simulink model "Xl_ch16_LPF_int_v6"  (Simulink 7.5)
settings: Solver=VariableStepDiscrete  StartTime=0.0  StopTime=0.001  RelTol=1e-3
values from neighbouring files (symbols this model uses):
  a2a = zeros(nFc, length(Hd.sosMatrix(:,5)))    [iirButter_SOS_init_v2.m]    (also in iirButter_SOS_init_v2_8pole.m)
  a3a = zeros(nFc, length(Hd.sosMatrix(:,6)))    [iirButter_SOS_init_v2.m]    (also in iirButter_SOS_init_v2_8pole.m)
  dt = 1/Fsim    (= 2.56e-06)    [iirButter_SOS_init_v2.m]    (also in iirButter_SOS_init_v2_8pole.m)
  Fc_min = 10    [iirButter_SOS_init_v2.m]    (also in iirButter_SOS_init_v2_8pole.m)
  ga = zeros(nFc, length(Hd.ScaleValues))    [iirButter_SOS_init_v2.m]    (also in iirButter_SOS_init_v2_8pole.m = zeros(nFc, length(Hd.ScaleValues(1:end-1))))
  rFc = (Fc_max/Fc_min)^(1/(nFc - 1))    (= 1.70532863139)    [iirButter_SOS_init_v2.m]    (also in iirButter_SOS_init_v2_8pole.m)
  Sra = 2^34|.02  |.027 |.027 |<.038| 1e-6|<2e-6|<2e-6|<2e-6|<2e-6| 8e-6|    [iirButter_SOS_init_v2.m]    (also in iirButter_SOS_init_v2_8pole.m)
  Srm = 2^34|     |     |     |     |     |     |     |     |     |  to |    [iirButter_SOS_init_v2.m]    (also in iirButter_SOS_init_v2_8pole.m)
libraries: xbsIndex_r4 x561, dspsrcs4 x16, simulink x8
(part 1 of 3)
CloseFcn:
  | rtwprivate ssgencode ModelCloseRequest Xl_ch16_LPF_int_v4
settings Model: Creator=Ivan  LastModifiedBy=val.fleyshman
settings OptimizationCC: InitFltsAndDblsToZero=on
settings DebuggingCC: SaveWithParameterizedLinksMsg=none  SignalResolutionControl=TryResolveAllWithWarning  StrictBusMsg=Warning
settings GRTTargetCC: TargetFcnLib=ansi_tfl_tmw.mat

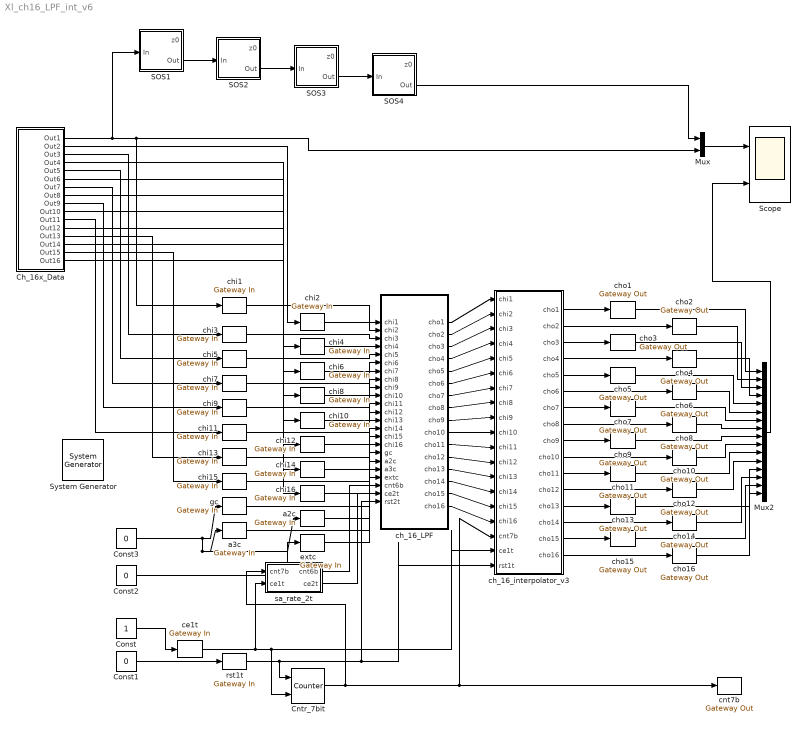
== system Xl_ch16_LPF_int_v6 ==
  " System Generator" : xbsIndex_r4/ System Generator  Tag=genX  SystemSampleTime=-1  xilinxfamily=spartan6  part=xc6slx45t  speed=-3  package=csg324  synthesis_tool=XST  clock_wrapper=Expose Clock Ports  directory=./netlist  testbench=off  simulink_period=1/50e6  sysclk_period=20  dcm_input_clock_period=10  incr_netlist=off  trim_vbits=Everywhere in SubSystem  dbl_ovrd=According to Block Masks  core_generation=According to Block Masks  run_coregen=off  deprecated_control=off  eval_field=0  block_type=sysgen
      settings: block_version=12.2
  Ch_16x_Data : Subsystem
  Cntr_7bit : xbsIndex_r4/Counter  cnt_type=Free Running  cnt_to=Inf  operation=Up  start_count=0  cnt_by_val=1  arith_type=Unsigned  n_bits=7  bin_pt=0  load_pin=off  rst=on  en=on  explicit_period=off  period=1/100e6  dbl_ovrd=off  use_behavioral_HDL=off  implementation=Fabric  block_type=counter
      settings: block_version=12.2
  Const : Constant  OutDataType=sfix(16)  OutScaling=2^0  SampleTime=dt / 128
  Const1 : Constant  Value=0  OutDataType=sfix(16)  OutScaling=2^0  SampleTime=dt / 128
  Const2 : Constant  Value=0  OutDataType=sfix(16)  OutScaling=2^0  SampleTime=dt / 128
  Const3 : Constant  Value=0  OutDataType=sfix(16)  OutScaling=2^0  SampleTime=dt / 128
  Mux : Mux  Inputs=2
  Mux2 : Mux  Inputs=16
  SOS1 : Subsystem
  SOS2 : Subsystem
  SOS3 : Subsystem
  SOS4 : Subsystem
  Scope : Scope  NumInputPorts=2
      settings: YMin=-1~-1  YMax=1~1  DataFormat=Structure  MaxDataPoints=5e6
  a2c : xbsIndex_r4/Gateway In  arith_type="Signed  (2's comp)"  n_bits=36  bin_pt=34  quantization=Truncate  overflow=Wrap  period=1/50e6  dbl_ovrd=off  timing_constraint=None  locs_specified=off  LOCs={}  hdl_port=on  block_type=gatewayin
      settings: infoedit="Gateway in block.  Converts inputs of type Simulink integer, double and fixed point to  Xilinx fixed point type.<br><br>Hardware notes:  In hardware these blocks become top level input ports."  block_version=12.2
  a3c : xbsIndex_r4/Gateway In  arith_type="Signed  (2's comp)"  n_bits=36  bin_pt=34  quantization=Truncate  overflow=Wrap  period=1/50e6  dbl_ovrd=off  timing_constraint=None  locs_specified=off  LOCs={}  hdl_port=on  block_type=gatewayin
      settings: infoedit="Gateway in block.  Converts inputs of type Simulink integer, double and fixed point to  Xilinx fixed point type.<br><br>Hardware notes:  In hardware these blocks become top level input ports."  block_version=12.2
  ce1t : xbsIndex_r4/Gateway In  arith_type=Boolean  n_bits=36  bin_pt=34  quantization=Truncate  overflow=Wrap  period=1/50e6  dbl_ovrd=off  timing_constraint=None  locs_specified=off  LOCs={}  hdl_port=on  block_type=gatewayin
      settings: infoedit="Gateway in block.  Converts inputs of type Simulink integer, double and fixed point to  Xilinx fixed point type.<br><br>Hardware notes:  In hardware these blocks become top level input ports."  block_version=12.2
  ch_16_LPF : Subsystem
  ch_16_interpolator_v3 : Subsystem
  chi{1..16} (16 alike) : xbsIndex_r4/Gateway In  arith_type="Signed  (2's comp)"  n_bits=18  bin_pt=16  quantization=Truncate  overflow=Wrap  period=1/50e6  dbl_ovrd=off  timing_constraint=None  locs_specified=off  LOCs={}  hdl_port=on  block_type=gatewayin
      settings: infoedit="Gateway in block.  Converts inputs of type Simulink integer, double and fixed point to  Xilinx fixed point type.<br><br>Hardware notes:  In hardware these blocks become top level input ports."  block_version=12.2
  cho{1..16} (16 alike) : xbsIndex_r4/Gateway Out  hdl_port=on  timing_constraint=None  locs_specified=off  LOCs={}  block_type=gatewayout
      settings: infoedit="Gateway out block.  Converts Xilinx fixed point inputs into ouputs of type Simulink integer, double, or fixed point.<br><br>Hardware notes:  In hardware these blocks become top level output ports or are discarded, depending on how they are configured."  block_version=12.2
  cnt7b : xbsIndex_r4/Gateway Out  hdl_port=on  timing_constraint=None  locs_specified=off  LOCs={}  block_type=gatewayout
      settings: infoedit="Gateway out block.  Converts Xilinx fixed point inputs into ouputs of type Simulink integer, double, or fixed point.<br><br>Hardware notes:  In hardware these blocks become top level output ports or are discarded, depending on how they are configured."  block_version=12.2
  extc : xbsIndex_r4/Gateway In  arith_type=Boolean  n_bits=36  bin_pt=34  quantization=Truncate  overflow=Wrap  period=1/50e6  dbl_ovrd=off  timing_constraint=None  locs_specified=off  LOCs={}  hdl_port=on  block_type=gatewayin
      settings: infoedit="Gateway in block.  Converts inputs of type Simulink integer, double and fixed point to  Xilinx fixed point type.<br><br>Hardware notes:  In hardware these blocks become top level input ports."  block_version=12.2
  gc : xbsIndex_r4/Gateway In  arith_type="Signed  (2's comp)"  n_bits=36  bin_pt=34  quantization=Truncate  overflow=Wrap  period=1/50e6  dbl_ovrd=off  timing_constraint=None  locs_specified=off  LOCs={}  hdl_port=on  block_type=gatewayin
      settings: infoedit="Gateway in block.  Converts inputs of type Simulink integer, double and fixed point to  Xilinx fixed point type.<br><br>Hardware notes:  In hardware these blocks become top level input ports."  block_version=12.2
  rst1t : xbsIndex_r4/Gateway In  arith_type=Boolean  n_bits=36  bin_pt=34  quantization=Truncate  overflow=Wrap  period=1/50e6  dbl_ovrd=off  timing_constraint=None  locs_specified=off  LOCs={}  hdl_port=on  block_type=gatewayin
      settings: infoedit="Gateway in block.  Converts inputs of type Simulink integer, double and fixed point to  Xilinx fixed point type.<br><br>Hardware notes:  In hardware these blocks become top level input ports."  block_version=12.2
  sa_rate_2t : Subsystem
  wires:
  SOS2/2(Out) -> SOS3/1(In)
  chi1/1 -> ch_16_LPF/1(chi1)
  chi2/1 -> ch_16_LPF/2(chi2)
  chi3/1 -> ch_16_LPF/3(chi3)
  chi4/1 -> ch_16_LPF/4(chi4)
  chi5/1 -> ch_16_LPF/5(chi5)
  chi6/1 -> ch_16_LPF/6(chi6)
  chi7/1 -> ch_16_LPF/7(chi7)
  chi8/1 -> ch_16_LPF/8(chi8)
  chi9/1 -> ch_16_LPF/9(chi9)
  chi10/1 -> ch_16_LPF/10(chi10)
  chi11/1 -> ch_16_LPF/11(chi11)
  chi12/1 -> ch_16_LPF/12(chi12)
  chi13/1 -> ch_16_LPF/13(chi13)
  chi14/1 -> ch_16_LPF/14(chi14)
  chi15/1 -> ch_16_LPF/15(chi15)
  chi16/1 -> ch_16_LPF/16(chi16)
  gc/1 -> ch_16_LPF/17(gc)
  a2c/1 -> ch_16_LPF/18(a2c)
  a3c/1 -> ch_16_LPF/19(a3c)
  ce1t/1 -> sa_rate_2t/2(ce1t), Cntr_7bit/2, ch_16_interpolator_v3/18(ce1t)
  rst1t/1 -> Cntr_7bit/1, ch_16_LPF/23(rst2t), ch_16_interpolator_v3/19(rst1t)
  Const1/1 -> rst1t/1
  sa_rate_2t/2(ce2t) -> ch_16_LPF/22(ce2t)
  extc/1 -> ch_16_LPF/20(extc)
  Const2/1 -> extc/1
  Const3/1 -> gc/1, a3c/1, a2c/1
  Cntr_7bit/1 -> sa_rate_2t/1(cnt7b), cnt7b/1, ch_16_interpolator_v3/17(cnt7b)
  sa_rate_2t/1(cnt6b) -> ch_16_LPF/21(cnt6b)
  Const/1 -> ce1t/1
  Mux/1 -> Scope/1
  SOS3/2(Out) -> SOS4/1(In)
  SOS1/2(Out) -> SOS2/1(In)
  SOS4/2(Out) -> Mux/1
  ch_16_interpolator_v3/1(cho1) -> cho1/1
  ch_16_interpolator_v3/2(cho2) -> cho2/1
  ch_16_interpolator_v3/3(cho3) -> cho3/1
  ch_16_interpolator_v3/4(cho4) -> cho4/1
  ch_16_interpolator_v3/5(cho5) -> cho5/1
  ch_16_interpolator_v3/6(cho6) -> cho6/1
  ch_16_interpolator_v3/7(cho7) -> cho7/1
  ch_16_interpolator_v3/8(cho8) -> cho8/1
  ch_16_interpolator_v3/9(cho9) -> cho9/1
  ch_16_interpolator_v3/10(cho10) -> cho10/1
  ch_16_interpolator_v3/11(cho11) -> cho11/1
  ch_16_interpolator_v3/12(cho12) -> cho12/1
  ch_16_interpolator_v3/13(cho13) -> cho13/1
  ch_16_interpolator_v3/14(cho14) -> cho14/1
  ch_16_interpolator_v3/15(cho15) -> cho15/1
  ch_16_interpolator_v3/16(cho16) -> cho16/1
  cho13/1 -> Mux2/13
  cho1/1 -> Mux2/1
  cho16/1 -> Mux2/16
  cho2/1 -> Mux2/2
  cho3/1 -> Mux2/3
  cho4/1 -> Mux2/4
  cho5/1 -> Mux2/5
  cho6/1 -> Mux2/6
  cho7/1 -> Mux2/7
  cho8/1 -> Mux2/8
  cho9/1 -> Mux2/9
  cho10/1 -> Mux2/10
  cho11/1 -> Mux2/11
  cho12/1 -> Mux2/12
  cho14/1 -> Mux2/14
  cho15/1 -> Mux2/15
  ch_16_LPF/1(cho1) -> ch_16_interpolator_v3/1(chi1)
  ch_16_LPF/2(cho2) -> ch_16_interpolator_v3/2(chi2)
  ch_16_LPF/3(cho3) -> ch_16_interpolator_v3/3(chi3)
  ch_16_LPF/4(cho4) -> ch_16_interpolator_v3/4(chi4)
  ch_16_LPF/5(cho5) -> ch_16_interpolator_v3/5(chi5)
  ch_16_LPF/6(cho6) -> ch_16_interpolator_v3/6(chi6)
  ch_16_LPF/7(cho7) -> ch_16_interpolator_v3/7(chi7)
  ch_16_LPF/8(cho8) -> ch_16_interpolator_v3/8(chi8)
  ch_16_LPF/9(cho9) -> ch_16_interpolator_v3/9(chi9)
  ch_16_LPF/10(cho10) -> ch_16_interpolator_v3/10(chi10)
  ch_16_LPF/11(cho11) -> ch_16_interpolator_v3/11(chi11)
  ch_16_LPF/12(cho12) -> ch_16_interpolator_v3/12(chi12)
  ch_16_LPF/13(cho13) -> ch_16_interpolator_v3/13(chi13)
  ch_16_LPF/14(cho14) -> ch_16_interpolator_v3/14(chi14)
  ch_16_LPF/15(cho15) -> ch_16_interpolator_v3/15(chi15)
  ch_16_LPF/16(cho16) -> ch_16_interpolator_v3/16(chi16)
  Mux2/1 -> Scope/2
  Ch_16x_Data/1(Out1) -> chi1/1, Mux/2, SOS1/1(In)
  Ch_16x_Data/2(Out2) -> chi2/1
  Ch_16x_Data/3(Out3) -> chi3/1
  Ch_16x_Data/4(Out4) -> chi4/1
  Ch_16x_Data/5(Out5) -> chi5/1
  Ch_16x_Data/6(Out6) -> chi6/1
  Ch_16x_Data/7(Out7) -> chi7/1
  Ch_16x_Data/8(Out8) -> chi8/1
  Ch_16x_Data/9(Out9) -> chi9/1
  Ch_16x_Data/10(Out10) -> chi10/1
  Ch_16x_Data/11(Out11) -> chi11/1
  Ch_16x_Data/12(Out12) -> chi12/1
  Ch_16x_Data/13(Out13) -> chi13/1
  Ch_16x_Data/14(Out14) -> chi14/1
  Ch_16x_Data/15(Out15) -> chi15/1
  Ch_16x_Data/16(Out16) -> chi16/1

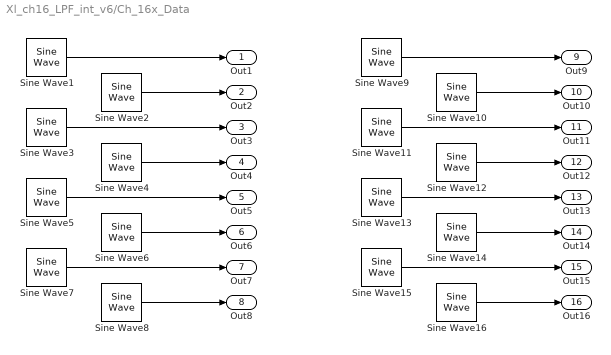
== system Xl_ch16_LPF_int_v6/Ch_16x_Data ==
  Sine Wave1 : dspsrcs4/Sine Wave  Amplitude=1  Frequency=Fc_min * rFc^(1 - 1)  Phase=0  SampleMode=Discrete  OutComplex=Real  CompMethod=Trigonometric fcn  TableSize=Speed  SampleTime=dt  SamplesPerFrame=1  dataType=double  wordLen=16  udDataType=sfix(16)  fracBitsMode=Best precision  numFracBits=15  ResetState=Restart at time zero
  Sine Wave10 : dspsrcs4/Sine Wave  Amplitude=1  Frequency=Fc_min * rFc^(10 - 1)  Phase=0  SampleMode=Discrete  OutComplex=Real  CompMethod=Trigonometric fcn  TableSize=Speed  SampleTime=dt  SamplesPerFrame=1  dataType=double  wordLen=16  udDataType=sfix(16)  fracBitsMode=Best precision  numFracBits=15  ResetState=Restart at time zero
  Sine Wave11 : dspsrcs4/Sine Wave  Amplitude=1  Frequency=Fc_min * rFc^(11 - 1)  Phase=0  SampleMode=Discrete  OutComplex=Real  CompMethod=Trigonometric fcn  TableSize=Speed  SampleTime=dt  SamplesPerFrame=1  dataType=double  wordLen=16  udDataType=sfix(16)  fracBitsMode=Best precision  numFracBits=15  ResetState=Restart at time zero
  Sine Wave12 : dspsrcs4/Sine Wave  Amplitude=1  Frequency=Fc_min * rFc^(12 - 1)  Phase=0  SampleMode=Discrete  OutComplex=Real  CompMethod=Trigonometric fcn  TableSize=Speed  SampleTime=dt  SamplesPerFrame=1  dataType=double  wordLen=16  udDataType=sfix(16)  fracBitsMode=Best precision  numFracBits=15  ResetState=Restart at time zero
  Sine Wave13 : dspsrcs4/Sine Wave  Amplitude=1  Frequency=Fc_min * rFc^(13 - 1)  Phase=0  SampleMode=Discrete  OutComplex=Real  CompMethod=Trigonometric fcn  TableSize=Speed  SampleTime=dt  SamplesPerFrame=1  dataType=double  wordLen=16  udDataType=sfix(16)  fracBitsMode=Best precision  numFracBits=15  ResetState=Restart at time zero
  Sine Wave14 : dspsrcs4/Sine Wave  Amplitude=1  Frequency=Fc_min * rFc^(14 - 1)  Phase=0  SampleMode=Discrete  OutComplex=Real  CompMethod=Trigonometric fcn  TableSize=Speed  SampleTime=dt  SamplesPerFrame=1  dataType=double  wordLen=16  udDataType=sfix(16)  fracBitsMode=Best precision  numFracBits=15  ResetState=Restart at time zero
  Sine Wave15 : dspsrcs4/Sine Wave  Amplitude=1  Frequency=Fc_min * rFc^(15 - 1)  Phase=0  SampleMode=Discrete  OutComplex=Real  CompMethod=Trigonometric fcn  TableSize=Speed  SampleTime=dt  SamplesPerFrame=1  dataType=double  wordLen=16  udDataType=sfix(16)  fracBitsMode=Best precision  numFracBits=15  ResetState=Restart at time zero
  Sine Wave16 : dspsrcs4/Sine Wave  Amplitude=1  Frequency=Fc_min * rFc^(16 - 1)  Phase=0  SampleMode=Discrete  OutComplex=Real  CompMethod=Trigonometric fcn  TableSize=Speed  SampleTime=dt  SamplesPerFrame=1  dataType=double  wordLen=16  udDataType=sfix(16)  fracBitsMode=Best precision  numFracBits=15  ResetState=Restart at time zero
  Sine Wave2 : dspsrcs4/Sine Wave  Amplitude=1  Frequency=Fc_min * rFc^(2 - 1)  Phase=0  SampleMode=Discrete  OutComplex=Real  CompMethod=Trigonometric fcn  TableSize=Speed  SampleTime=dt  SamplesPerFrame=1  dataType=double  wordLen=16  udDataType=sfix(16)  fracBitsMode=Best precision  numFracBits=15  ResetState=Restart at time zero
  Sine Wave3 : dspsrcs4/Sine Wave  Amplitude=1  Frequency=Fc_min * rFc^(3 - 1)  Phase=0  SampleMode=Discrete  OutComplex=Real  CompMethod=Trigonometric fcn  TableSize=Speed  SampleTime=dt  SamplesPerFrame=1  dataType=double  wordLen=16  udDataType=sfix(16)  fracBitsMode=Best precision  numFracBits=15  ResetState=Restart at time zero
  Sine Wave4 : dspsrcs4/Sine Wave  Amplitude=1  Frequency=Fc_min * rFc^(4 - 1)  Phase=0  SampleMode=Discrete  OutComplex=Real  CompMethod=Trigonometric fcn  TableSize=Speed  SampleTime=dt  SamplesPerFrame=1  dataType=double  wordLen=16  udDataType=sfix(16)  fracBitsMode=Best precision  numFracBits=15  ResetState=Restart at time zero
  Sine Wave5 : dspsrcs4/Sine Wave  Amplitude=1  Frequency=Fc_min * rFc^(5 - 1)  Phase=0  SampleMode=Discrete  OutComplex=Real  CompMethod=Trigonometric fcn  TableSize=Speed  SampleTime=dt  SamplesPerFrame=1  dataType=double  wordLen=16  udDataType=sfix(16)  fracBitsMode=Best precision  numFracBits=15  ResetState=Restart at time zero
  Sine Wave6 : dspsrcs4/Sine Wave  Amplitude=1  Frequency=Fc_min * rFc^(6 - 1)  Phase=0  SampleMode=Discrete  OutComplex=Real  CompMethod=Trigonometric fcn  TableSize=Speed  SampleTime=dt  SamplesPerFrame=1  dataType=double  wordLen=16  udDataType=sfix(16)  fracBitsMode=Best precision  numFracBits=15  ResetState=Restart at time zero
  Sine Wave7 : dspsrcs4/Sine Wave  Amplitude=1  Frequency=Fc_min * rFc^(7 - 1)  Phase=0  SampleMode=Discrete  OutComplex=Real  CompMethod=Trigonometric fcn  TableSize=Speed  SampleTime=dt  SamplesPerFrame=1  dataType=double  wordLen=16  udDataType=sfix(16)  fracBitsMode=Best precision  numFracBits=15  ResetState=Restart at time zero
  Sine Wave8 : dspsrcs4/Sine Wave  Amplitude=1  Frequency=Fc_min * rFc^(8 - 1)  Phase=0  SampleMode=Discrete  OutComplex=Real  CompMethod=Trigonometric fcn  TableSize=Speed  SampleTime=dt  SamplesPerFrame=1  dataType=double  wordLen=16  udDataType=sfix(16)  fracBitsMode=Best precision  numFracBits=15  ResetState=Restart at time zero
  Sine Wave9 : dspsrcs4/Sine Wave  Amplitude=1  Frequency=Fc_min * rFc^(9 - 1)  Phase=0  SampleMode=Discrete  OutComplex=Real  CompMethod=Trigonometric fcn  TableSize=Speed  SampleTime=dt  SamplesPerFrame=1  dataType=double  wordLen=16  udDataType=sfix(16)  fracBitsMode=Best precision  numFracBits=15  ResetState=Restart at time zero
  Out1 : Outport
  Out2 : Outport  Port=2
  Out3 : Outport  Port=3
  Out4 : Outport  Port=4
  Out5 : Outport  Port=5
  Out6 : Outport  Port=6
  Out7 : Outport  Port=7
  Out8 : Outport  Port=8
  Out9 : Outport  Port=9
  Out10 : Outport  Port=10
  Out11 : Outport  Port=11
  Out12 : Outport  Port=12
  Out13 : Outport  Port=13
  Out14 : Outport  Port=14
  Out15 : Outport  Port=15
  Out16 : Outport  Port=16
  wires:
  Sine Wave16/1 -> Out16/1
  Sine Wave15/1 -> Out15/1
  Sine Wave14/1 -> Out14/1
  Sine Wave13/1 -> Out13/1
  Sine Wave12/1 -> Out12/1
  Sine Wave11/1 -> Out11/1
  Sine Wave10/1 -> Out10/1
  Sine Wave9/1 -> Out9/1
  Sine Wave8/1 -> Out8/1
  Sine Wave7/1 -> Out7/1
  Sine Wave6/1 -> Out6/1
  Sine Wave5/1 -> Out5/1
  Sine Wave4/1 -> Out4/1
  Sine Wave3/1 -> Out3/1
  Sine Wave2/1 -> Out2/1
  Sine Wave1/1 -> Out1/1

== system Xl_ch16_LPF_int_v6/SOS1 ==
  note: b1 = 1
  note: b3 = 1
  note: 1/a1 = 1
  In : Inport
  Delay : simulink/Discrete/Integer Delay  vinit=0.0  samptime=-1  NumDelays=1
  Delay1 : simulink/Discrete/Integer Delay  vinit=0.0  samptime=-1  NumDelays=1
  Round RA : Subsystem
  Round RA1 : Subsystem
  Round RM : Subsystem
  Round RM1 : Subsystem
  Round RM2 : Subsystem
  Sum Denom1 : Sum  Inputs=+-  OutDataType=sfix(16)  OutScaling=2^0
  Sum Denom2 : Sum  Inputs=+-  OutDataType=sfix(16)  OutScaling=2^0
  Sum Num1 : Sum  OutDataType=sfix(16)  OutScaling=2^0
  Sum Num2 : Sum  OutDataType=sfix(16)  OutScaling=2^0
  a2 : Gain  Gain=a2a(13,1)  ParameterDataType=sfix(16)  ParameterScaling=2^0  OutDataType=sfix(16)  OutScaling=2^0
  a3 : Gain  Gain=a3a(13,1)  ParameterDataType=sfix(16)  ParameterScaling=2^0  OutDataType=sfix(16)  OutScaling=2^0
  b2 : Gain  Gain=2  ParameterDataType=sfix(16)  ParameterScaling=2^0  OutDataType=sfix(16)  OutScaling=2^0
  g : Gain  Gain=ga(13,1)  ParameterDataType=sfix(16)  ParameterScaling=2^0  OutDataType=sfix(16)  OutScaling=2^0
  z0 : Outport
  Out : Outport  Port=2
  wires:
  Delay/1 -> Delay1/1, b2/1, a2/1
  b2/1 -> Sum Num1/2
  Delay1/1 -> a3/1, Sum Num2/2
  Sum Denom2/1 -> Round RA/1(In)
  a2/1 -> Round RM1/1(In)
  a3/1 -> Round RM2/1(In)
  g/1 -> Round RM/1(In)
  In/1 -> g/1
  Sum Num2/1 -> Round RA1/1(In)
  Round RM/1(Out) -> Sum Denom1/1
  Round RA/1(Out) -> Delay/1, z0/1, Sum Num1/1
  Round RA1/1(Out) -> Out/1
  Sum Num1/1 -> Sum Num2/1
  Sum Denom1/1 -> Sum Denom2/1
  Round RM1/1(Out) -> Sum Denom1/2
  Round RM2/1(Out) -> Sum Denom2/2

== system Xl_ch16_LPF_int_v6/SOS2 ==
  note: 1/a1 = 1
  note: b3 = 1
  note: b1 = 1
  In : Inport
  Delay : simulink/Discrete/Integer Delay  vinit=0.0  samptime=-1  NumDelays=1
  Delay1 : simulink/Discrete/Integer Delay  vinit=0.0  samptime=-1  NumDelays=1
  Round RA : Subsystem
  Round RA1 : Subsystem
  Round RM : Subsystem
  Round RM1 : Subsystem
  Round RM2 : Subsystem
  Sum Denom1 : Sum  Inputs=+-  OutDataType=sfix(16)  OutScaling=2^0
  Sum Denom2 : Sum  Inputs=+-  OutDataType=sfix(16)  OutScaling=2^0
  Sum Num1 : Sum  OutDataType=sfix(16)  OutScaling=2^0
  Sum Num2 : Sum  OutDataType=sfix(16)  OutScaling=2^0
  a2 : Gain  Gain=a2a(13,2)  ParameterDataType=sfix(16)  ParameterScaling=2^0  OutDataType=sfix(16)  OutScaling=2^0
  a3 : Gain  Gain=a3a(13,2)  ParameterDataType=sfix(16)  ParameterScaling=2^0  OutDataType=sfix(16)  OutScaling=2^0
  b2 : Gain  Gain=2  ParameterDataType=sfix(16)  ParameterScaling=2^0  OutDataType=sfix(16)  OutScaling=2^0
  g : Gain  Gain=ga(13,2)  ParameterDataType=sfix(16)  ParameterScaling=2^0  OutDataType=sfix(16)  OutScaling=2^0
  z0 : Outport
  Out : Outport  Port=2
  wires:
  Round RM2/1(Out) -> Sum Denom2/2
  Round RM1/1(Out) -> Sum Denom1/2
  Sum Denom1/1 -> Sum Denom2/1
  Sum Num1/1 -> Sum Num2/1
  Round RA1/1(Out) -> Out/1
  Round RA/1(Out) -> Sum Num1/1, z0/1, Delay/1
  Round RM/1(Out) -> Sum Denom1/1
  Sum Num2/1 -> Round RA1/1(In)
  In/1 -> g/1
  g/1 -> Round RM/1(In)
  a3/1 -> Round RM2/1(In)
  a2/1 -> Round RM1/1(In)
  Sum Denom2/1 -> Round RA/1(In)
  Delay1/1 -> Sum Num2/2, a3/1
  b2/1 -> Sum Num1/2
  Delay/1 -> a2/1, b2/1, Delay1/1

== system Xl_ch16_LPF_int_v6/SOS3 ==
  note: b1 = 1
  note: b3 = 1
  note: 1/a1 = 1
  In : Inport
  Delay : simulink/Discrete/Integer Delay  vinit=0.0  samptime=-1  NumDelays=1
  Delay1 : simulink/Discrete/Integer Delay  vinit=0.0  samptime=-1  NumDelays=1
  Round RA : Subsystem
  Round RA1 : Subsystem
  Round RM : Subsystem
  Round RM1 : Subsystem
  Round RM2 : Subsystem
  Sum Denom1 : Sum  Inputs=+-  OutDataType=sfix(16)  OutScaling=2^0
  Sum Denom2 : Sum  Inputs=+-  OutDataType=sfix(16)  OutScaling=2^0
  Sum Num1 : Sum  OutDataType=sfix(16)  OutScaling=2^0
  Sum Num2 : Sum  OutDataType=sfix(16)  OutScaling=2^0
  a2 : Gain  Gain=a2a(13,3)  ParameterDataType=sfix(16)  ParameterScaling=2^0  OutDataType=sfix(16)  OutScaling=2^0
  a3 : Gain  Gain=a3a(13,3)  ParameterDataType=sfix(16)  ParameterScaling=2^0  OutDataType=sfix(16)  OutScaling=2^0
  b2 : Gain  Gain=2  ParameterDataType=sfix(16)  ParameterScaling=2^0  OutDataType=sfix(16)  OutScaling=2^0
  g : Gain  Gain=ga(13,3)  ParameterDataType=sfix(16)  ParameterScaling=2^0  OutDataType=sfix(16)  OutScaling=2^0
  z0 : Outport
  Out : Outport  Port=2
  wires:
  Delay/1 -> Delay1/1, b2/1, a2/1
  b2/1 -> Sum Num1/2
  Delay1/1 -> a3/1, Sum Num2/2
  Sum Denom2/1 -> Round RA/1(In)
  a2/1 -> Round RM1/1(In)
  a3/1 -> Round RM2/1(In)
  g/1 -> Round RM/1(In)
  In/1 -> g/1
  Sum Num2/1 -> Round RA1/1(In)
  Round RM/1(Out) -> Sum Denom1/1
  Round RA/1(Out) -> Delay/1, z0/1, Sum Num1/1
  Round RA1/1(Out) -> Out/1
  Sum Num1/1 -> Sum Num2/1
  Sum Denom1/1 -> Sum Denom2/1
  Round RM1/1(Out) -> Sum Denom1/2
  Round RM2/1(Out) -> Sum Denom2/2

== system Xl_ch16_LPF_int_v6/SOS4 ==
  note: b1 = 1
  note: b3 = 1
  note: 1/a1 = 1
  In : Inport
  Delay : simulink/Discrete/Integer Delay  vinit=0.0  samptime=-1  NumDelays=1
  Delay1 : simulink/Discrete/Integer Delay  vinit=0.0  samptime=-1  NumDelays=1
  Round RA : Subsystem
  Round RA1 : Subsystem
  Round RM : Subsystem
  Round RM1 : Subsystem
  Round RM2 : Subsystem
  Sum Denom1 : Sum  Inputs=+-  OutDataType=sfix(16)  OutScaling=2^0
  Sum Denom2 : Sum  Inputs=+-  OutDataType=sfix(16)  OutScaling=2^0
  Sum Num1 : Sum  OutDataType=sfix(16)  OutScaling=2^0
  Sum Num2 : Sum  OutDataType=sfix(16)  OutScaling=2^0
  a2 : Gain  Gain=a2a(13,4)  ParameterDataType=sfix(16)  ParameterScaling=2^0  OutDataType=sfix(16)  OutScaling=2^0
  a3 : Gain  Gain=a3a(13,4)  ParameterDataType=sfix(16)  ParameterScaling=2^0  OutDataType=sfix(16)  OutScaling=2^0
  b2 : Gain  Gain=2  ParameterDataType=sfix(16)  ParameterScaling=2^0  OutDataType=sfix(16)  OutScaling=2^0
  g : Gain  Gain=ga(13,4)  ParameterDataType=sfix(16)  ParameterScaling=2^0  OutDataType=sfix(16)  OutScaling=2^0
  z0 : Outport
  Out : Outport  Port=2
  wires:
  Delay/1 -> Delay1/1, b2/1, a2/1
  b2/1 -> Sum Num1/2
  Delay1/1 -> a3/1, Sum Num2/2
  Sum Denom2/1 -> Round RA/1(In)
  a2/1 -> Round RM1/1(In)
  a3/1 -> Round RM2/1(In)
  g/1 -> Round RM/1(In)
  In/1 -> g/1
  Sum Num2/1 -> Round RA1/1(In)
  Round RM/1(Out) -> Sum Denom1/1
  Round RA/1(Out) -> Delay/1, z0/1, Sum Num1/1
  Round RA1/1(Out) -> Out/1
  Sum Num1/1 -> Sum Num2/1
  Sum Denom1/1 -> Sum Denom2/1
  Round RM1/1(Out) -> Sum Denom1/2
  Round RM2/1(Out) -> Sum Denom2/2

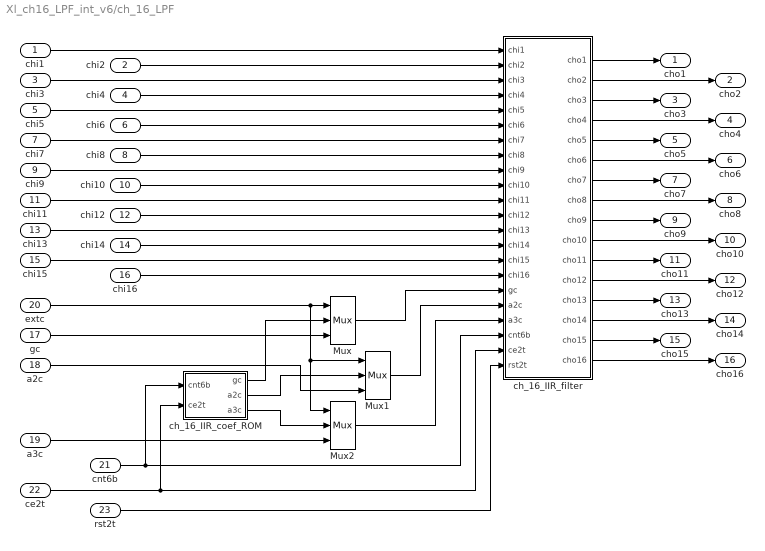
== system Xl_ch16_LPF_int_v6/ch_16_LPF ==
  chi1 : Inport
  chi2 : Inport  Port=2
  chi3 : Inport  Port=3
  chi4 : Inport  Port=4
  chi5 : Inport  Port=5
  chi6 : Inport  Port=6
  chi7 : Inport  Port=7
  chi8 : Inport  Port=8
  chi9 : Inport  Port=9
  chi10 : Inport  Port=10
  chi11 : Inport  Port=11
  chi12 : Inport  Port=12
  chi13 : Inport  Port=13
  chi14 : Inport  Port=14
  chi15 : Inport  Port=15
  chi16 : Inport  Port=16
  gc : Inport  Port=17
  a2c : Inport  Port=18
  a3c : Inport  Port=19
  extc : Inport  Port=20
  cnt6b : Inport  Port=21
  ce2t : Inport  Port=22
  rst2t : Inport  Port=23
  Mux : xbsIndex_r4/Mux  inputs=2  en=off  latency=0  precision=Full  arith_type=Unsigned  n_bits=16  bin_pt=14  quantization=Truncate  overflow=Wrap  dbl_ovrd=off  block_type=mux
      settings: block_version=12.2
  Mux1 : xbsIndex_r4/Mux  inputs=2  en=off  latency=0  precision=Full  arith_type=Unsigned  n_bits=16  bin_pt=14  quantization=Truncate  overflow=Wrap  dbl_ovrd=off  block_type=mux
      settings: block_version=12.2
  Mux2 : xbsIndex_r4/Mux  inputs=2  en=off  latency=0  precision=Full  arith_type=Unsigned  n_bits=16  bin_pt=14  quantization=Truncate  overflow=Wrap  dbl_ovrd=off  block_type=mux
      settings: block_version=12.2
  ch_16_IIR_coef_ROM : Subsystem
  ch_16_IIR_filter : Subsystem
  cho1 : Outport
  cho2 : Outport  Port=2
  cho3 : Outport  Port=3
  cho4 : Outport  Port=4
  cho5 : Outport  Port=5
  cho6 : Outport  Port=6
  cho7 : Outport  Port=7
  cho8 : Outport  Port=8
  cho9 : Outport  Port=9
  cho10 : Outport  Port=10
  cho11 : Outport  Port=11
  cho12 : Outport  Port=12
  cho13 : Outport  Port=13
  cho14 : Outport  Port=14
  cho15 : Outport  Port=15
  cho16 : Outport  Port=16
  wires:
  chi1/1 -> ch_16_IIR_filter/1(chi1)
  ch_16_IIR_filter/1(cho1) -> cho1/1
  chi2/1 -> ch_16_IIR_filter/2(chi2)
  ch_16_IIR_filter/2(cho2) -> cho2/1
  chi3/1 -> ch_16_IIR_filter/3(chi3)
  ch_16_IIR_filter/3(cho3) -> cho3/1
  chi4/1 -> ch_16_IIR_filter/4(chi4)
  chi5/1 -> ch_16_IIR_filter/5(chi5)
  ch_16_IIR_filter/4(cho4) -> cho4/1
  chi6/1 -> ch_16_IIR_filter/6(chi6)
  ch_16_IIR_filter/5(cho5) -> cho5/1
  chi7/1 -> ch_16_IIR_filter/7(chi7)
  ch_16_IIR_filter/6(cho6) -> cho6/1
  chi8/1 -> ch_16_IIR_filter/8(chi8)
  chi9/1 -> ch_16_IIR_filter/9(chi9)
  ch_16_IIR_filter/7(cho7) -> cho7/1
  chi10/1 -> ch_16_IIR_filter/10(chi10)
  ch_16_IIR_filter/8(cho8) -> cho8/1
  chi11/1 -> ch_16_IIR_filter/11(chi11)
  ch_16_IIR_filter/9(cho9) -> cho9/1
  chi12/1 -> ch_16_IIR_filter/12(chi12)
  chi13/1 -> ch_16_IIR_filter/13(chi13)
  ch_16_IIR_filter/10(cho10) -> cho10/1
  chi14/1 -> ch_16_IIR_filter/14(chi14)
  ch_16_IIR_filter/11(cho11) -> cho11/1
  chi15/1 -> ch_16_IIR_filter/15(chi15)
  ch_16_IIR_filter/12(cho12) -> cho12/1
  chi16/1 -> ch_16_IIR_filter/16(chi16)
  ch_16_IIR_filter/13(cho13) -> cho13/1
  ch_16_IIR_filter/14(cho14) -> cho14/1
  ch_16_IIR_filter/15(cho15) -> cho15/1
  ce2t/1 -> ch_16_IIR_coef_ROM/2(ce2t), ch_16_IIR_filter/21(ce2t)
  ch_16_IIR_filter/16(cho16) -> cho16/1
  gc/1 -> Mux/3
  Mux/1 -> ch_16_IIR_filter/17(gc)
  a2c/1 -> Mux1/3
  Mux1/1 -> ch_16_IIR_filter/18(a2c)
  Mux2/1 -> ch_16_IIR_filter/19(a3c)
  a3c/1 -> Mux2/3
  extc/1 -> Mux/1, Mux2/1, Mux1/1
  ch_16_IIR_coef_ROM/1(gc) -> Mux/2
  ch_16_IIR_coef_ROM/3(a3c) -> Mux2/2
  rst2t/1 -> ch_16_IIR_filter/22(rst2t)
  cnt6b/1 -> ch_16_IIR_coef_ROM/1(cnt6b), ch_16_IIR_filter/20(cnt6b)
  ch_16_IIR_coef_ROM/2(a2c) -> Mux1/2

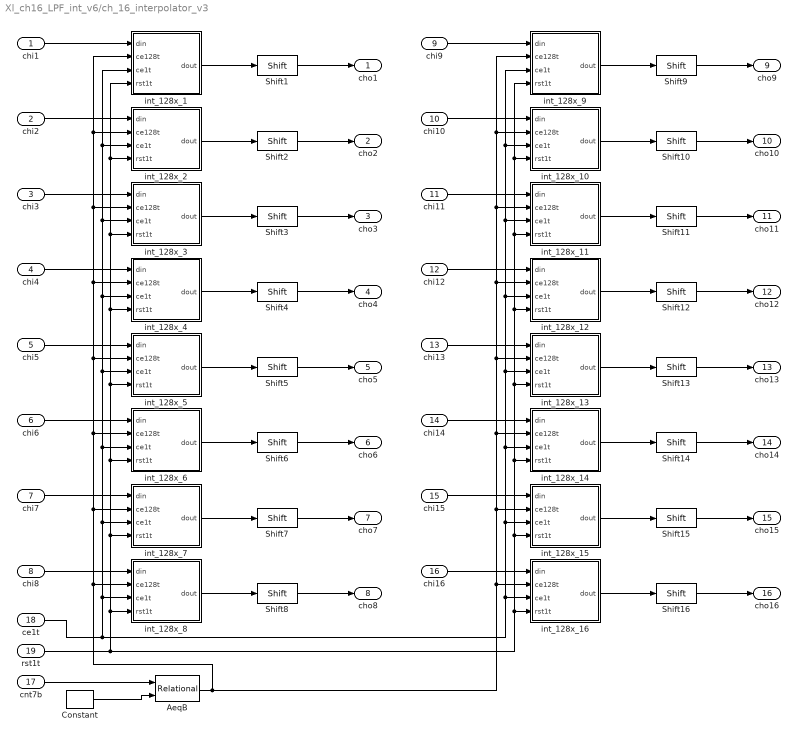
== system Xl_ch16_LPF_int_v6/ch_16_interpolator_v3 ==
  chi1 : Inport
  chi2 : Inport  Port=2
  chi3 : Inport  Port=3
  chi4 : Inport  Port=4
  chi5 : Inport  Port=5
  chi6 : Inport  Port=6
  chi7 : Inport  Port=7
  chi8 : Inport  Port=8
  chi9 : Inport  Port=9
  chi10 : Inport  Port=10
  chi11 : Inport  Port=11
  chi12 : Inport  Port=12
  chi13 : Inport  Port=13
  chi14 : Inport  Port=14
  chi15 : Inport  Port=15
  chi16 : Inport  Port=16
  cnt7b : Inport  Port=17
  ce1t : Inport  Port=18
  rst1t : Inport  Port=19
  AeqB : xbsIndex_r4/Relational  mode=a=b  en=off  latency=0  dbl_ovrd=off  block_type=relational
      settings: block_version=12.2
  Constant : xbsIndex_r4/Constant  arith_type=Unsigned  const=0  n_bits=7  bin_pt=0  explicit_period=off  period=1  equ=P=C  opselect=C  inp2=PCIN>>17  opr=+  inp1=P  carry=CIN  dbl_ovrd=off  block_type=constant
      settings: block_version=12.2
  Shift{1..16} (16 alike) : xbsIndex_r4/Shift  shift_dir=Right  shift_bits=14  en=off  latency=0  precision=User Defined  arith_type="Signed  (2's comp)"  n_bits=18  bin_pt=16  quantization=Truncate  overflow=Wrap  dbl_ovrd=off  block_type=shift
      settings: xl_area=[0 0 0 0 0 0 0]  block_version=12.2
  int_128x_1 : Subsystem
  int_128x_10 : Subsystem
  int_128x_11 : Subsystem
  int_128x_12 : Subsystem
  int_128x_13 : Subsystem
  int_128x_14 : Subsystem
  int_128x_15 : Subsystem
  int_128x_16 : Subsystem
  int_128x_2 : Subsystem
  int_128x_3 : Subsystem
  int_128x_4 : Subsystem
  int_128x_5 : Subsystem
  int_128x_6 : Subsystem
  int_128x_7 : Subsystem
  int_128x_8 : Subsystem
  int_128x_9 : Subsystem
  cho1 : Outport
  cho2 : Outport  Port=2
  cho3 : Outport  Port=3
  cho4 : Outport  Port=4
  cho5 : Outport  Port=5
  cho6 : Outport  Port=6
  cho7 : Outport  Port=7
  cho8 : Outport  Port=8
  cho9 : Outport  Port=9
  cho10 : Outport  Port=10
  cho11 : Outport  Port=11
  cho12 : Outport  Port=12
  cho13 : Outport  Port=13
  cho14 : Outport  Port=14
  cho15 : Outport  Port=15
  cho16 : Outport  Port=16
  wires:
  int_128x_1/1(dout) -> Shift1/1
  chi1/1 -> int_128x_1/1(din)
  Shift1/1 -> cho1/1
  int_128x_2/1(dout) -> Shift2/1
  chi2/1 -> int_128x_2/1(din)
  Shift2/1 -> cho2/1
  int_128x_3/1(dout) -> Shift3/1
  chi3/1 -> int_128x_3/1(din)
  Shift3/1 -> cho3/1
  int_128x_4/1(dout) -> Shift4/1
  chi4/1 -> int_128x_4/1(din)
  Shift4/1 -> cho4/1
  int_128x_5/1(dout) -> Shift5/1
  chi5/1 -> int_128x_5/1(din)
  Shift5/1 -> cho5/1
  int_128x_6/1(dout) -> Shift6/1
  chi6/1 -> int_128x_6/1(din)
  Shift6/1 -> cho6/1
  int_128x_7/1(dout) -> Shift7/1
  chi7/1 -> int_128x_7/1(din)
  Shift7/1 -> cho7/1
  int_128x_8/1(dout) -> Shift8/1
  chi8/1 -> int_128x_8/1(din)
  Shift8/1 -> cho8/1
  int_128x_9/1(dout) -> Shift9/1
  chi9/1 -> int_128x_9/1(din)
  Shift9/1 -> cho9/1
  int_128x_10/1(dout) -> Shift10/1
  chi10/1 -> int_128x_10/1(din)
  Shift10/1 -> cho10/1
  int_128x_11/1(dout) -> Shift11/1
  chi11/1 -> int_128x_11/1(din)
  Shift11/1 -> cho11/1
  int_128x_12/1(dout) -> Shift12/1
  chi12/1 -> int_128x_12/1(din)
  Shift12/1 -> cho12/1
  int_128x_13/1(dout) -> Shift13/1
  chi13/1 -> int_128x_13/1(din)
  Shift13/1 -> cho13/1
  int_128x_14/1(dout) -> Shift14/1
  chi14/1 -> int_128x_14/1(din)
  Shift14/1 -> cho14/1
  int_128x_15/1(dout) -> Shift15/1
  chi15/1 -> int_128x_15/1(din)
  Shift15/1 -> cho15/1
  int_128x_16/1(dout) -> Shift16/1
  chi16/1 -> int_128x_16/1(din)
  Shift16/1 -> cho16/1
  rst1t/1 -> int_128x_1/4(rst1t), int_128x_2/4(rst1t), int_128x_3/4(rst1t), int_128x_4/4(rst1t), int_128x_5/4(rst1t), int_128x_6/4(rst1t), int_128x_7/4(rst1t), int_128x_8/4(rst1t), int_128x_9/4(rst1t), int_128x_10/4(rst1t), int_128x_11/4(rst1t), int_128x_12/4(rst1t), int_128x_13/4(rst1t), int_128x_14/4(rst1t), int_128x_15/4(rst1t), int_128x_16/4(rst1t)
  ce1t/1 -> int_128x_1/3(ce1t), int_128x_2/3(ce1t), int_128x_3/3(ce1t), int_128x_4/3(ce1t), int_128x_5/3(ce1t), int_128x_6/3(ce1t), int_128x_7/3(ce1t), int_128x_8/3(ce1t), int_128x_9/3(ce1t), int_128x_10/3(ce1t), int_128x_11/3(ce1t), int_128x_12/3(ce1t), int_128x_13/3(ce1t), int_128x_14/3(ce1t), int_128x_15/3(ce1t), int_128x_16/3(ce1t)
  AeqB/1 -> int_128x_1/2(ce128t), int_128x_2/2(ce128t), int_128x_3/2(ce128t), int_128x_4/2(ce128t), int_128x_5/2(ce128t), int_128x_6/2(ce128t), int_128x_7/2(ce128t), int_128x_8/2(ce128t), int_128x_9/2(ce128t), int_128x_10/2(ce128t), int_128x_11/2(ce128t), int_128x_12/2(ce128t), int_128x_13/2(ce128t), int_128x_14/2(ce128t), int_128x_15/2(ce128t), int_128x_16/2(ce128t)
  cnt7b/1 -> AeqB/1
  Constant/1 -> AeqB/2

== system Xl_ch16_LPF_int_v6/sa_rate_2t ==
  cnt7b : Inport
  ce1t : Inport  Port=2
  Extract_LSB : xbsIndex_r4/Slice  nbits=1  boolean_output=on  mode=Lower Bit Location + Width  bit1=0  base1=MSB of Input  bit0=0  base0=LSB of Input  dbl_ovrd=off  block_type=slice
      settings: block_version=12.2
  Logical : xbsIndex_r4/Logical  logical_function=AND  inputs=2  en=off  latency=0  precision=Full  arith_type=Unsigned  n_bits=16  bin_pt=0  align_bp=on  dbl_ovrd=off  block_type=logical
      settings: block_version=12.2
  Slice_6MSB : xbsIndex_r4/Slice  nbits=6  boolean_output=off  mode=Upper Bit Location + Width  bit1=0  base1=MSB of Input  bit0=0  base0=LSB of Input  dbl_ovrd=off  block_type=slice
      settings: block_version=12.2
  cnt6b : Outport
  ce2t : Outport  Port=2
  wires:
  cnt7b/1 -> Slice_6MSB/1, Extract_LSB/1
  Slice_6MSB/1 -> cnt6b/1
  Extract_LSB/1 -> Logical/1
  Logical/1 -> ce2t/1
  ce1t/1 -> Logical/2

== system Xl_ch16_LPF_int_v6/SOS1/Round RA ==
  In : Inport
  Rounding Function : Rounding  Operator=round
  Scale Back : Gain  Gain=1/Sra  ParameterDataType=sfix(16)  ParameterScaling=2^0  OutDataType=sfix(16)  OutScaling=2^0
  Scale Up : Gain  Gain=Sra  ParameterDataType=sfix(16)  ParameterScaling=2^0  OutDataType=sfix(16)  OutScaling=2^0
  Out : Outport
  wires:
  Scale Back/1 -> Out/1
  In/1 -> Scale Up/1
  Rounding Function/1 -> Scale Back/1
  Scale Up/1 -> Rounding Function/1

== system Xl_ch16_LPF_int_v6/SOS1/Round RA1 ==
  In : Inport
  Rounding Function : Rounding  Operator=round
  Scale Back : Gain  Gain=1/Sra  ParameterDataType=sfix(16)  ParameterScaling=2^0  OutDataType=sfix(16)  OutScaling=2^0
  Scale Up : Gain  Gain=Sra  ParameterDataType=sfix(16)  ParameterScaling=2^0  OutDataType=sfix(16)  OutScaling=2^0
  Out : Outport
  wires:
  Scale Up/1 -> Rounding Function/1
  Rounding Function/1 -> Scale Back/1
  In/1 -> Scale Up/1
  Scale Back/1 -> Out/1

== system Xl_ch16_LPF_int_v6/SOS1/Round RM ==
  In : Inport
  Rounding Function : Rounding  Operator=round
  Scale Back : Gain  Gain=1/Srm  ParameterDataType=sfix(16)  ParameterScaling=2^0  OutDataType=sfix(16)  OutScaling=2^0
  Scale Up : Gain  Gain=Srm  ParameterDataType=sfix(16)  ParameterScaling=2^0  OutDataType=sfix(16)  OutScaling=2^0
  Out : Outport
  wires:
  Scale Up/1 -> Rounding Function/1
  Rounding Function/1 -> Scale Back/1
  In/1 -> Scale Up/1
  Scale Back/1 -> Out/1

== system Xl_ch16_LPF_int_v6/SOS1/Round RM1 ==
  In : Inport
  Rounding Function : Rounding  Operator=round
  Scale Back : Gain  Gain=1/Srm  ParameterDataType=sfix(16)  ParameterScaling=2^0  OutDataType=sfix(16)  OutScaling=2^0
  Scale Up : Gain  Gain=Srm  ParameterDataType=sfix(16)  ParameterScaling=2^0  OutDataType=sfix(16)  OutScaling=2^0
  Out : Outport
  wires:
  Scale Back/1 -> Out/1
  In/1 -> Scale Up/1
  Rounding Function/1 -> Scale Back/1
  Scale Up/1 -> Rounding Function/1

== system Xl_ch16_LPF_int_v6/SOS1/Round RM2 ==
  In : Inport
  Rounding Function : Rounding  Operator=round
  Scale Back : Gain  Gain=1/Srm  ParameterDataType=sfix(16)  ParameterScaling=2^0  OutDataType=sfix(16)  OutScaling=2^0
  Scale Up : Gain  Gain=Srm  ParameterDataType=sfix(16)  ParameterScaling=2^0  OutDataType=sfix(16)  OutScaling=2^0
  Out : Outport
  wires:
  Scale Up/1 -> Rounding Function/1
  Rounding Function/1 -> Scale Back/1
  In/1 -> Scale Up/1
  Scale Back/1 -> Out/1

== system Xl_ch16_LPF_int_v6/SOS2/Round RA ==
  In : Inport
  Rounding Function : Rounding  Operator=round
  Scale Back : Gain  Gain=1/Sra  ParameterDataType=sfix(16)  ParameterScaling=2^0  OutDataType=sfix(16)  OutScaling=2^0
  Scale Up : Gain  Gain=Sra  ParameterDataType=sfix(16)  ParameterScaling=2^0  OutDataType=sfix(16)  OutScaling=2^0
  Out : Outport
  wires:
  Scale Up/1 -> Rounding Function/1
  Rounding Function/1 -> Scale Back/1
  In/1 -> Scale Up/1
  Scale Back/1 -> Out/1

== system Xl_ch16_LPF_int_v6/SOS2/Round RA1 ==
  In : Inport
  Rounding Function : Rounding  Operator=round
  Scale Back : Gain  Gain=1/Sra  ParameterDataType=sfix(16)  ParameterScaling=2^0  OutDataType=sfix(16)  OutScaling=2^0
  Scale Up : Gain  Gain=Sra  ParameterDataType=sfix(16)  ParameterScaling=2^0  OutDataType=sfix(16)  OutScaling=2^0
  Out : Outport
  wires:
  Scale Back/1 -> Out/1
  In/1 -> Scale Up/1
  Rounding Function/1 -> Scale Back/1
  Scale Up/1 -> Rounding Function/1

== system Xl_ch16_LPF_int_v6/SOS2/Round RM ==
  In : Inport
  Rounding Function : Rounding  Operator=round
  Scale Back : Gain  Gain=1/Srm  ParameterDataType=sfix(16)  ParameterScaling=2^0  OutDataType=sfix(16)  OutScaling=2^0
  Scale Up : Gain  Gain=Srm  ParameterDataType=sfix(16)  ParameterScaling=2^0  OutDataType=sfix(16)  OutScaling=2^0
  Out : Outport
  wires:
  Scale Back/1 -> Out/1
  In/1 -> Scale Up/1
  Rounding Function/1 -> Scale Back/1
  Scale Up/1 -> Rounding Function/1

== system Xl_ch16_LPF_int_v6/SOS2/Round RM1 ==
  In : Inport
  Rounding Function : Rounding  Operator=round
  Scale Back : Gain  Gain=1/Srm  ParameterDataType=sfix(16)  ParameterScaling=2^0  OutDataType=sfix(16)  OutScaling=2^0
  Scale Up : Gain  Gain=Srm  ParameterDataType=sfix(16)  ParameterScaling=2^0  OutDataType=sfix(16)  OutScaling=2^0
  Out : Outport
  wires:
  Scale Up/1 -> Rounding Function/1
  Rounding Function/1 -> Scale Back/1
  In/1 -> Scale Up/1
  Scale Back/1 -> Out/1

== system Xl_ch16_LPF_int_v6/SOS2/Round RM2 ==
  In : Inport
  Rounding Function : Rounding  Operator=round
  Scale Back : Gain  Gain=1/Srm  ParameterDataType=sfix(16)  ParameterScaling=2^0  OutDataType=sfix(16)  OutScaling=2^0
  Scale Up : Gain  Gain=Srm  ParameterDataType=sfix(16)  ParameterScaling=2^0  OutDataType=sfix(16)  OutScaling=2^0
  Out : Outport
  wires:
  Scale Back/1 -> Out/1
  In/1 -> Scale Up/1
  Rounding Function/1 -> Scale Back/1
  Scale Up/1 -> Rounding Function/1

== system Xl_ch16_LPF_int_v6/SOS3/Round RA ==
  In : Inport
  Rounding Function : Rounding  Operator=round
  Scale Back : Gain  Gain=1/Sra  ParameterDataType=sfix(16)  ParameterScaling=2^0  OutDataType=sfix(16)  OutScaling=2^0
  Scale Up : Gain  Gain=Sra  ParameterDataType=sfix(16)  ParameterScaling=2^0  OutDataType=sfix(16)  OutScaling=2^0
  Out : Outport
  wires:
  Scale Back/1 -> Out/1
  In/1 -> Scale Up/1
  Rounding Function/1 -> Scale Back/1
  Scale Up/1 -> Rounding Function/1

== system Xl_ch16_LPF_int_v6/SOS3/Round RA1 ==
  In : Inport
  Rounding Function : Rounding  Operator=round
  Scale Back : Gain  Gain=1/Sra  ParameterDataType=sfix(16)  ParameterScaling=2^0  OutDataType=sfix(16)  OutScaling=2^0
  Scale Up : Gain  Gain=Sra  ParameterDataType=sfix(16)  ParameterScaling=2^0  OutDataType=sfix(16)  OutScaling=2^0
  Out : Outport
  wires:
  Scale Up/1 -> Rounding Function/1
  Rounding Function/1 -> Scale Back/1
  In/1 -> Scale Up/1
  Scale Back/1 -> Out/1

== system Xl_ch16_LPF_int_v6/SOS3/Round RM ==
  In : Inport
  Rounding Function : Rounding  Operator=round
  Scale Back : Gain  Gain=1/Srm  ParameterDataType=sfix(16)  ParameterScaling=2^0  OutDataType=sfix(16)  OutScaling=2^0
  Scale Up : Gain  Gain=Srm  ParameterDataType=sfix(16)  ParameterScaling=2^0  OutDataType=sfix(16)  OutScaling=2^0
  Out : Outport
  wires:
  Scale Up/1 -> Rounding Function/1
  Rounding Function/1 -> Scale Back/1
  In/1 -> Scale Up/1
  Scale Back/1 -> Out/1

== system Xl_ch16_LPF_int_v6/SOS3/Round RM1 ==
  In : Inport
  Rounding Function : Rounding  Operator=round
  Scale Back : Gain  Gain=1/Srm  ParameterDataType=sfix(16)  ParameterScaling=2^0  OutDataType=sfix(16)  OutScaling=2^0
  Scale Up : Gain  Gain=Srm  ParameterDataType=sfix(16)  ParameterScaling=2^0  OutDataType=sfix(16)  OutScaling=2^0
  Out : Outport
  wires:
  Scale Back/1 -> Out/1
  In/1 -> Scale Up/1
  Rounding Function/1 -> Scale Back/1
  Scale Up/1 -> Rounding Function/1

== system Xl_ch16_LPF_int_v6/SOS3/Round RM2 ==
  In : Inport
  Rounding Function : Rounding  Operator=round
  Scale Back : Gain  Gain=1/Srm  ParameterDataType=sfix(16)  ParameterScaling=2^0  OutDataType=sfix(16)  OutScaling=2^0
  Scale Up : Gain  Gain=Srm  ParameterDataType=sfix(16)  ParameterScaling=2^0  OutDataType=sfix(16)  OutScaling=2^0
  Out : Outport
  wires:
  Scale Up/1 -> Rounding Function/1
  Rounding Function/1 -> Scale Back/1
  In/1 -> Scale Up/1
  Scale Back/1 -> Out/1

== system Xl_ch16_LPF_int_v6/SOS4/Round RA ==
  In : Inport
  Rounding Function : Rounding  Operator=round
  Scale Back : Gain  Gain=1/Sra  ParameterDataType=sfix(16)  ParameterScaling=2^0  OutDataType=sfix(16)  OutScaling=2^0
  Scale Up : Gain  Gain=Sra  ParameterDataType=sfix(16)  ParameterScaling=2^0  OutDataType=sfix(16)  OutScaling=2^0
  Out : Outport
  wires:
  Scale Back/1 -> Out/1
  In/1 -> Scale Up/1
  Rounding Function/1 -> Scale Back/1
  Scale Up/1 -> Rounding Function/1

== system Xl_ch16_LPF_int_v6/SOS4/Round RA1 ==
  In : Inport
  Rounding Function : Rounding  Operator=round
  Scale Back : Gain  Gain=1/Sra  ParameterDataType=sfix(16)  ParameterScaling=2^0  OutDataType=sfix(16)  OutScaling=2^0
  Scale Up : Gain  Gain=Sra  ParameterDataType=sfix(16)  ParameterScaling=2^0  OutDataType=sfix(16)  OutScaling=2^0
  Out : Outport
  wires:
  Scale Up/1 -> Rounding Function/1
  Rounding Function/1 -> Scale Back/1
  In/1 -> Scale Up/1
  Scale Back/1 -> Out/1

== system Xl_ch16_LPF_int_v6/SOS4/Round RM ==
  In : Inport
  Rounding Function : Rounding  Operator=round
  Scale Back : Gain  Gain=1/Srm  ParameterDataType=sfix(16)  ParameterScaling=2^0  OutDataType=sfix(16)  OutScaling=2^0
  Scale Up : Gain  Gain=Srm  ParameterDataType=sfix(16)  ParameterScaling=2^0  OutDataType=sfix(16)  OutScaling=2^0
  Out : Outport
  wires:
  Scale Up/1 -> Rounding Function/1
  Rounding Function/1 -> Scale Back/1
  In/1 -> Scale Up/1
  Scale Back/1 -> Out/1

== system Xl_ch16_LPF_int_v6/SOS4/Round RM1 ==
  In : Inport
  Rounding Function : Rounding  Operator=round
  Scale Back : Gain  Gain=1/Srm  ParameterDataType=sfix(16)  ParameterScaling=2^0  OutDataType=sfix(16)  OutScaling=2^0
  Scale Up : Gain  Gain=Srm  ParameterDataType=sfix(16)  ParameterScaling=2^0  OutDataType=sfix(16)  OutScaling=2^0
  Out : Outport
  wires:
  Scale Back/1 -> Out/1
  In/1 -> Scale Up/1
  Rounding Function/1 -> Scale Back/1
  Scale Up/1 -> Rounding Function/1

== system Xl_ch16_LPF_int_v6/SOS4/Round RM2 ==
  In : Inport
  Rounding Function : Rounding  Operator=round
  Scale Back : Gain  Gain=1/Srm  ParameterDataType=sfix(16)  ParameterScaling=2^0  OutDataType=sfix(16)  OutScaling=2^0
  Scale Up : Gain  Gain=Srm  ParameterDataType=sfix(16)  ParameterScaling=2^0  OutDataType=sfix(16)  OutScaling=2^0
  Out : Outport
  wires:
  Scale Up/1 -> Rounding Function/1
  Rounding Function/1 -> Scale Back/1
  In/1 -> Scale Up/1
  Scale Back/1 -> Out/1

== system Xl_ch16_LPF_int_v6/ch_16_LPF/ch_16_IIR_coef_ROM ==
  cnt6b : Inport
  ce2t : Inport  Port=2
  a2c_ROM : xbsIndex_r4/ROM  depth=64  initVector=a2_16x4x  distributed_mem=Block RAM  rst=off  init_reg=0  en=on  latency=2  arith_type="Signed  (2's comp)"  n_bits=36  bin_pt=34  dbl_ovrd=off  optimize=Area  use_rpm=on  block_type=sprom
      settings: block_version=12.2
  a3c_ROM : xbsIndex_r4/ROM  depth=64  initVector=a3_16x4x  distributed_mem=Block RAM  rst=off  init_reg=0  en=on  latency=2  arith_type="Signed  (2's comp)"  n_bits=36  bin_pt=34  dbl_ovrd=off  optimize=Area  use_rpm=on  block_type=sprom
      settings: block_version=12.2
  gc_ROM : xbsIndex_r4/ROM  depth=64  initVector=g_16x4x  distributed_mem=Block RAM  rst=off  init_reg=0  en=on  latency=2  arith_type="Signed  (2's comp)"  n_bits=36  bin_pt=34  dbl_ovrd=off  optimize=Area  use_rpm=on  block_type=sprom
      settings: block_version=12.2
  gc : Outport
  a2c : Outport  Port=2
  a3c : Outport  Port=3
  wires:
  cnt6b/1 -> a3c_ROM/1, a2c_ROM/1, gc_ROM/1
  ce2t/1 -> a2c_ROM/2, gc_ROM/2, a3c_ROM/2
  a3c_ROM/1 -> a3c/1
  a2c_ROM/1 -> a2c/1
  gc_ROM/1 -> gc/1

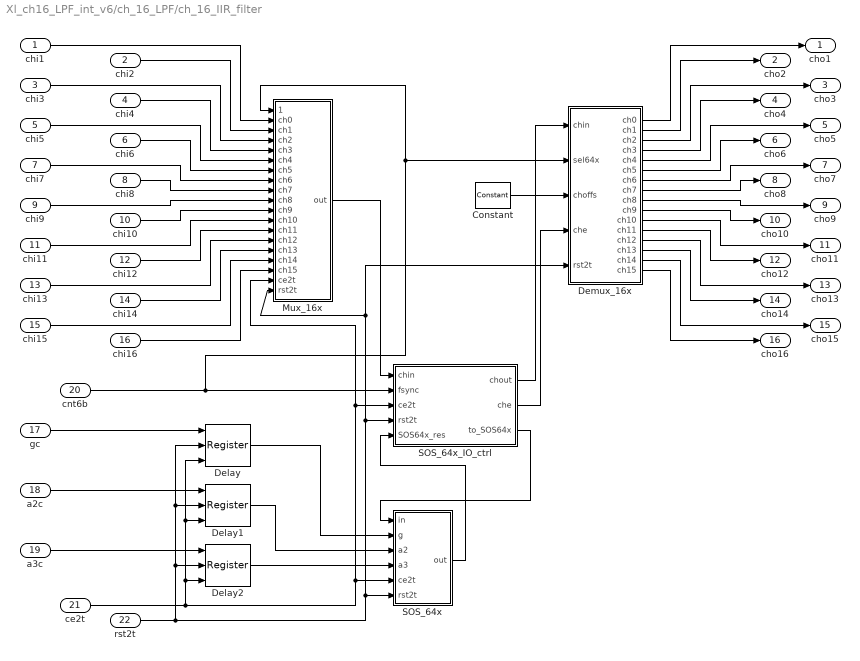
== system Xl_ch16_LPF_int_v6/ch_16_LPF/ch_16_IIR_filter ==
  chi1 : Inport  OutDataType=fixdt(1, 16)  OutScaling=2^0
  chi2 : Inport  Port=2  OutDataType=fixdt(1, 16)  OutScaling=2^0
  chi3 : Inport  Port=3  OutDataType=fixdt(1, 16)  OutScaling=2^0
  chi4 : Inport  Port=4  OutDataType=fixdt(1, 16)  OutScaling=2^0
  chi5 : Inport  Port=5  OutDataType=fixdt(1, 16)  OutScaling=2^0
  chi6 : Inport  Port=6  OutDataType=fixdt(1, 16)  OutScaling=2^0
  chi7 : Inport  Port=7  OutDataType=fixdt(1, 16)  OutScaling=2^0
  chi8 : Inport  Port=8  OutDataType=fixdt(1, 16)  OutScaling=2^0
  chi9 : Inport  Port=9  OutDataType=fixdt(1, 16)  OutScaling=2^0
  chi10 : Inport  Port=10  OutDataType=fixdt(1, 16)  OutScaling=2^0
  chi11 : Inport  Port=11  OutDataType=fixdt(1, 16)  OutScaling=2^0
  chi12 : Inport  Port=12  OutDataType=fixdt(1, 16)  OutScaling=2^0
  chi13 : Inport  Port=13  OutDataType=fixdt(1, 16)  OutScaling=2^0
  chi14 : Inport  Port=14  OutDataType=fixdt(1, 16)  OutScaling=2^0
  chi15 : Inport  Port=15  OutDataType=fixdt(1, 16)  OutScaling=2^0
  chi16 : Inport  Port=16  OutDataType=fixdt(1, 16)  OutScaling=2^0
  gc : Inport  Port=17  OutDataType=fixdt(1, 16)  OutScaling=2^0
  a2c : Inport  Port=18  OutDataType=fixdt(1, 16)  OutScaling=2^0
  a3c : Inport  Port=19  OutDataType=fixdt(1, 16)  OutScaling=2^0
  cnt6b : Inport  Port=20  OutDataType=fixdt(1, 16)  OutScaling=2^0
  ce2t : Inport  Port=21  OutDataType=fixdt(1, 16)  OutScaling=2^0
  rst2t : Inport  Port=22  OutDataType=fixdt(1, 16)  OutScaling=2^0
  Constant : xbsIndex_r4/Constant  arith_type=Unsigned  const=14  n_bits=4  bin_pt=0  explicit_period=off  period=1  equ=P=C  opselect=C  inp2=PCIN>>17  opr=+  inp1=P  carry=CIN  dbl_ovrd=off  block_type=constant
      settings: block_version=12.2
  Delay : xbsIndex_r4/Register  init=0  rst=on  en=on  dbl_ovrd=off  block_type=register
      settings: block_version=12.2
  Delay1 : xbsIndex_r4/Register  init=0  rst=on  en=on  dbl_ovrd=off  block_type=register
      settings: block_version=12.2
  Delay2 : xbsIndex_r4/Register  init=0  rst=on  en=on  dbl_ovrd=off  block_type=register
      settings: block_version=12.2
  Demux_16x : Subsystem
  Mux_16x : Subsystem
  SOS_64x : Subsystem
  SOS_64x_IO_ctrl : Subsystem
  cho1 : Outport  OutDataType=fixdt(1, 16)  OutScaling=2^0
  cho2 : Outport  Port=2  OutDataType=fixdt(1, 16)  OutScaling=2^0
  cho3 : Outport  Port=3  OutDataType=fixdt(1, 16)  OutScaling=2^0
  cho4 : Outport  Port=4  OutDataType=fixdt(1, 16)  OutScaling=2^0
  cho5 : Outport  Port=5  OutDataType=fixdt(1, 16)  OutScaling=2^0
  cho6 : Outport  Port=6  OutDataType=fixdt(1, 16)  OutScaling=2^0
  cho7 : Outport  Port=7  OutDataType=fixdt(1, 16)  OutScaling=2^0
  cho8 : Outport  Port=8  OutDataType=fixdt(1, 16)  OutScaling=2^0
  cho9 : Outport  Port=9  OutDataType=fixdt(1, 16)  OutScaling=2^0
  cho10 : Outport  Port=10  OutDataType=fixdt(1, 16)  OutScaling=2^0
  cho11 : Outport  Port=11  OutDataType=fixdt(1, 16)  OutScaling=2^0
  cho12 : Outport  Port=12  OutDataType=fixdt(1, 16)  OutScaling=2^0
  cho13 : Outport  Port=13  OutDataType=fixdt(1, 16)  OutScaling=2^0
  cho14 : Outport  Port=14  OutDataType=fixdt(1, 16)  OutScaling=2^0
  cho15 : Outport  Port=15  OutDataType=fixdt(1, 16)  OutScaling=2^0
  cho16 : Outport  Port=16  OutDataType=fixdt(1, 16)  OutScaling=2^0
  wires:
  gc/1 -> Delay/1
  a2c/1 -> Delay1/1
  a3c/1 -> Delay2/1
  ce2t/1 -> Delay/3, Delay1/3, Delay2/3, SOS_64x/5(ce2t), SOS_64x_IO_ctrl/3(ce2t), Mux_16x/18(ce2t)
  rst2t/1 -> Delay/2, Delay1/2, Delay2/2, SOS_64x/6(rst2t), SOS_64x_IO_ctrl/4(rst2t), Demux_16x/5(rst2t), Mux_16x/19(rst2t)
  SOS_64x_IO_ctrl/3(to_SOS64x) -> SOS_64x/1(in)
  SOS_64x/1(out) -> SOS_64x_IO_ctrl/5(SOS64x_res)
  SOS_64x_IO_ctrl/1(chout) -> Demux_16x/1(chin)
  Constant/1 -> Demux_16x/3(choffs)
  Delay/1 -> SOS_64x/2(g)
  Delay1/1 -> SOS_64x/3(a2)
  Delay2/1 -> SOS_64x/4(a3)
  chi8/1 -> Mux_16x/9(ch7)
  chi9/1 -> Mux_16x/10(ch8)
  chi7/1 -> Mux_16x/8(ch6)
  chi6/1 -> Mux_16x/7(ch5)
  chi5/1 -> Mux_16x/6(ch4)
  chi4/1 -> Mux_16x/5(ch3)
  chi3/1 -> Mux_16x/4(ch2)
  chi2/1 -> Mux_16x/3(ch1)
  chi1/1 -> Mux_16x/2(ch0)
  chi10/1 -> Mux_16x/11(ch9)
  chi11/1 -> Mux_16x/12(ch10)
  chi12/1 -> Mux_16x/13(ch11)
  chi13/1 -> Mux_16x/14(ch12)
  chi14/1 -> Mux_16x/15(ch13)
  chi15/1 -> Mux_16x/16(ch14)
  chi16/1 -> Mux_16x/17(ch15)
  Demux_16x/8(ch7) -> cho8/1
  Demux_16x/9(ch8) -> cho9/1
  Demux_16x/7(ch6) -> cho7/1
  Demux_16x/6(ch5) -> cho6/1
  Demux_16x/5(ch4) -> cho5/1
  Demux_16x/4(ch3) -> cho4/1
  Demux_16x/3(ch2) -> cho3/1
  Demux_16x/2(ch1) -> cho2/1
  Demux_16x/1(ch0) -> cho1/1
  Demux_16x/10(ch9) -> cho10/1
  Demux_16x/11(ch10) -> cho11/1
  Demux_16x/12(ch11) -> cho12/1
  Demux_16x/13(ch12) -> cho13/1
  Demux_16x/14(ch13) -> cho14/1
  Demux_16x/15(ch14) -> cho15/1
  Demux_16x/16(ch15) -> cho16/1
  cnt6b/1 -> SOS_64x_IO_ctrl/2(fsync), Demux_16x/2(sel64x), Mux_16x/1(sel64x)
  Mux_16x/1(out) -> SOS_64x_IO_ctrl/1(chin)
  SOS_64x_IO_ctrl/2(che) -> Demux_16x/4(che)
